simulink model "New_model_FOPID"  (R2016a)
settings: Solver=VariableStepAuto  StartTime=0.0  StopTime=50  RelTol=1e-3
undefined symbols (not defined in the file or in its folder): kk
libraries: fod x3
settings Model: Creator=EBUKA  LastModifiedBy=EBUKA
settings GRTTargetCC: GeneratePreprocessorConditionals=Use local settings

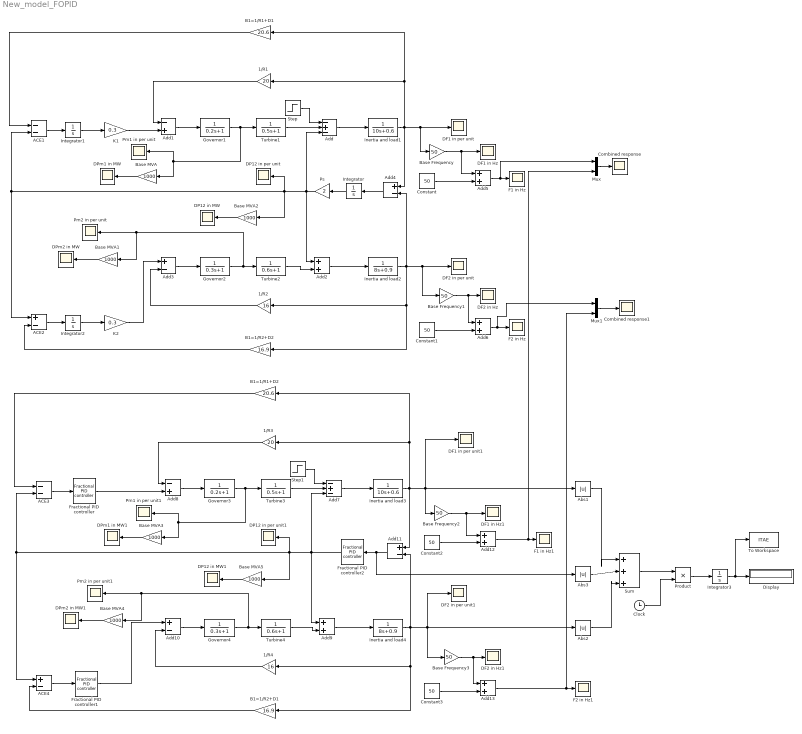
== system New_model_FOPID ==
  1/R1 : Gain  Gain=20
  1/R2 : Gain  Gain=16
  1/R3 : Gain  Gain=20
  1/R4 : Gain  Gain=16
  ACE1 : Sum  Inputs=--
  ACE2 : Sum  Inputs=+-
  ACE3 : Sum  Inputs=--
  ACE4 : Sum  Inputs=+-
  Abs1 : Abs
  Abs2 : Abs
  Abs3 : Abs
  Add : Sum  Inputs=-+-
  Add1 : Sum  Inputs=-+
  Add{3..4,10..11} (4 alike) : Sum  Inputs=+-
  Add{2,5..6,9,12..13} (6 alike) : Sum
  Add7 : Sum  Inputs=-+-
  Add8 : Sum  Inputs=-+
  B1=1/R1+D1 : Gain  Gain=20.6
  B1=1/R1+D2 : Gain  Gain=20.6
  B1=1/R2+D1 : Gain  Gain=16.9
  B1=1/R2+D2 : Gain  Gain=16.9
  Base Frequency{,1..3} (4 alike) : Gain  Gain=50
  Base MVA{,1..5} (6 alike) : Gain  Gain=1000
  Clock : Clock
  Combined response : Scope
  Combined response1 : Scope
  Constant{,1..3} (4 alike) : Constant  Value=50
  DF1 in Hz : Scope
  DF1 in Hz1 : Scope
  DF1 in per unit : Scope
  DF1 in per unit1 : Scope
  DF2 in Hz : Scope
  DF2 in Hz1 : Scope
  DF2 in per unit : Scope
  DF2 in per unit1 : Scope
  DP12 in MW : Scope
  DP12 in MW1 : Scope
  DP12 in per unit : Scope
  DP12 in per unit1 : Scope
  DPm1 in MW : Scope
  DPm1 in MW1 : Scope
  DPm2 in MW : Scope
  DPm2 in MW1 : Scope
  Display : Display
  F1 in Hz : Scope
  F1 in Hz1 : Scope
  F2 in Hz : Scope
  F2 in Hz1 : Scope
  Fractional PID controller : fod/Fractional PID controller  Kp=kk(1)  Ki=kk(2)  lambda=kk(10)  Kd=kk(3)  mic=kk(11)  freqRange=[0.001, 1000]  N=5
      link override Derivative Gain: Gain=kk(3)
      link override Fractional derivative1/Transfer Fcn1: Denominator=[kk(11) 1]
      link override Fractional integrator1/Transfer Fcn1: Denominator=[kk(10) 1]
      link override Integral Gain: Gain=kk(2)
      link override Proportional Gain: Gain=kk(1)
  Fractional PID controller1 : fod/Fractional PID controller  Kp=kk(4)  Ki=kk(5)  lambda=kk(12)  Kd=kk(6)  mic=kk(13)  freqRange=[0.001, 1000]  N=5
      link override Derivative Gain: Gain=kk(6)
      link override Fractional derivative1/Transfer Fcn1: Denominator=[kk(13) 1]
      link override Fractional integrator1/Transfer Fcn1: Denominator=[kk(12) 1]
      link override Integral Gain: Gain=kk(5)
      link override Proportional Gain: Gain=kk(4)
  Fractional PID controller2 : fod/Fractional PID controller  Kp=kk(7)  Ki=kk(8)  lambda=kk(14)  Kd=kk(9)  mic=kk(15)  freqRange=[0.001, 1000]  N=5
      link override Derivative Gain: Gain=kk(9)
      link override Fractional derivative1/Transfer Fcn1: Denominator=[kk(15) 1]
      link override Fractional integrator1/Transfer Fcn1: Denominator=[kk(14) 1]
      link override Integral Gain: Gain=kk(8)
      link override Proportional Gain: Gain=kk(7)
  Governor1 : TransferFcn  Denominator=[0.2 1]
  Governor2 : TransferFcn  Denominator=[0.3 1]
  Governor3 : TransferFcn  Denominator=[0.2 1]
  Governor4 : TransferFcn  Denominator=[0.3 1]
  Inertia and load1 : TransferFcn  Denominator=[10 0.6]
  Inertia and load2 : TransferFcn  Denominator=[8 0.9]
  Inertia and load3 : TransferFcn  Denominator=[10 0.6]
  Inertia and load4 : TransferFcn  Denominator=[8 0.9]
  Integrator{,1..3} (4 alike) : Integrator
  K1 : Gain  Gain=0.3
  K2 : Gain  Gain=0.3
  Mux : Mux  Inputs=2
  Mux1 : Mux  Inputs=2
  Pm1 in per unit : Scope
  Pm1 in per unit1 : Scope
  Pm2 in per unit : Scope
  Pm2 in per unit1 : Scope
  Product : Product
  Ps : Gain  Gain=2
  Step : Step  Time=100  Before=0.1  After=0.1  SampleTime=0
  Step1 : Step  Time=100  Before=0.1  After=0.1  SampleTime=0
  Sum : Sum  Inputs=|+++
  To Workspace : ToWorkspace  VariableName=ITAE  SampleTime=-1
  Turbine1 : TransferFcn  Denominator=[0.5 1]
  Turbine2 : TransferFcn  Denominator=[0.6 1]
  Turbine3 : TransferFcn  Denominator=[0.5 1]
  Turbine4 : TransferFcn  Denominator=[0.6 1]
  wires:
  Add/1 -> Inertia and load1/1
  Turbine1/1 -> Add/2
  Governor1/1 -> Base MVA/1, Pm1 in per unit/1, Turbine1/1
  Add1/1 -> Governor1/1
  1/R1/1 -> Add1/1
  Add2/1 -> Inertia and load2/1
  Turbine2/1 -> Add2/2
  Add3/1 -> Governor2/1
  Add4/1 -> Integrator/1
  Integrator/1 -> Ps/1
  Step/1 -> Add/1
  Base Frequency/1 -> Add5/1, DF1 in Hz/1
  Base Frequency1/1 -> Add6/1, DF2 in Hz/1
  Constant/1 -> Add5/2
  Add5/1 -> Mux/1, F1 in Hz/1
  Constant1/1 -> Add6/2
  Add6/1 -> Mux1/1, F2 in Hz/1
  Base MVA/1 -> DPm1 in MW/1
  Governor2/1 -> Pm2 in per unit/1, Base MVA1/1, Turbine2/1
  Base MVA1/1 -> DPm2 in MW/1
  Ps/1 -> ACE2/1, ACE1/2, Base MVA2/1, DP12 in per unit/1, Add2/1, Add/3
  Base MVA2/1 -> DP12 in MW/1
  Inertia and load1/1 -> Add4/1, Base Frequency/1, DF1 in per unit/1, B1=1/R1+D1/1, 1/R1/1
  B1=1/R1+D1/1 -> ACE1/1
  Integrator1/1 -> K1/1
  K1/1 -> Add1/2
  ACE1/1 -> Integrator1/1
  Inertia and load2/1 -> Base Frequency1/1, DF2 in per unit/1, Add4/2, B1=1/R2+D2/1, 1/R2/1
  B1=1/R2+D2/1 -> ACE2/2
  Integrator2/1 -> K2/1
  K2/1 -> Add3/1
  ACE2/1 -> Integrator2/1
  1/R2/1 -> Add3/2
  Add7/1 -> Inertia and load3/1
  Turbine3/1 -> Add7/2
  Governor3/1 -> Base MVA3/1, Pm1 in per unit1/1, Turbine3/1
  Add8/1 -> Governor3/1
  1/R3/1 -> Add8/1
  Add9/1 -> Inertia and load4/1
  Turbine4/1 -> Add9/2
  Add10/1 -> Governor4/1
  Step1/1 -> Add7/1
  Base Frequency2/1 -> Add12/1, DF1 in Hz1/1
  Base Frequency3/1 -> Add13/1, DF2 in Hz1/1
  Constant2/1 -> Add12/2
  Constant3/1 -> Add13/2
  Base MVA3/1 -> DPm1 in MW1/1
  Governor4/1 -> Pm2 in per unit1/1, Base MVA4/1, Turbine4/1
  Base MVA4/1 -> DPm2 in MW1/1
  Fractional PID controller2/1 -> ACE4/1, ACE3/2, Base MVA5/1, DP12 in per unit1/1, Add9/1, Add7/3
  Base MVA5/1 -> DP12 in MW1/1
  Inertia and load3/1 -> Add11/1, Abs1/1, Base Frequency2/1, DF1 in per unit1/1, B1=1/R1+D2/1, 1/R3/1
  B1=1/R1+D2/1 -> ACE3/1
  Fractional PID controller/1 -> Add8/2
  ACE3/1 -> Fractional PID controller/1
  Inertia and load4/1 -> Base Frequency3/1, Abs2/1, DF2 in per unit1/1, Add11/2, B1=1/R2+D1/1, 1/R4/1
  B1=1/R2+D1/1 -> ACE4/2
  Fractional PID controller1/1 -> Add10/1
  1/R4/1 -> Add10/2
  ACE4/1 -> Fractional PID controller1/1
  Add11/1 -> Fractional PID controller2/1, Abs3/1
  Add12/1 -> Mux/2, F1 in Hz1/1
  Mux/1 -> Combined response/1
  Mux1/1 -> Combined response1/1
  Add13/1 -> Mux1/2, F2 in Hz1/1
  Abs1/1 -> Sum/1
  Abs3/1 -> Sum/2
  Abs2/1 -> Sum/3
  Sum/1 -> Product/1
  Clock/1 -> Product/2
  Product/1 -> Integrator3/1
  Integrator3/1 -> To Workspace/1, Display/1
